simulink model "vehicle_suspension_model"  (R2015b)
settings: Solver=ode45  SolverMode=SingleTasking  StartTime=0.0  StopTime=10  MaxStep=0.01  RelTol=1e-3  AbsTol=1e-6
StopFcn:
  | if exist('sldemo_suspn_output')
  | sldemo_suspgraph
  | end
model workspace (MATLAB code in the model file):
  | sldemo_suspdat; %load data from file
undefined symbols (not defined in the file or in its folder): Iyy, Mb
undefined symbols (not defined in the file): cf, cr, kf, kr, Lf, Lr
CloseFcn:
  | if exist('suspnFigH')
  |   if ishghandle(suspnFigH,'figure')
  |     close(suspnFigH)
  |   end
  |   clear suspnFigH
  | end
  | if exist('suspnAxH'), clear suspnAxH; end
Description:
  | Automotive Suspension
  | 
  | This example shows how to model a simplified half-car model that includes an independent
  | front and rear vertical suspension. The model also includes body pitch and
  | bounce degrees of freedom. The example provides a description of the model to
  | show how simulation can be used for investigating ride characteristics.
  | In conjunction with a powertrain simulation, the model could
  | investigate longitudinal shuffle resulting from changes in throttle setting.
settings Model: ExtModeTrigMode=oneshot  ExtModeArmWhenConnect=off  ExtModeAutoUpdateStatusClock=off  Creator=The MathWorks, Inc.  LastModifiedBy=Samuel
settings DataIOCC: InitialState=x0  LimitDataPoints=off  SaveFormat=StructureWithTime  SaveOutput=off  SaveTime=off  StateSaveName=x  TimeSaveName=t  SignalLoggingName=sldemo_suspn_output
settings OptimizationCC: ExpressionDepthLimit=2147483647  InitFltsAndDblsToZero=on  BufferReusableBoundary=off
settings DebuggingCC: SaveWithParameterizedLinksMsg=none  UnderspecifiedInitializationDetection=Classic  MergeDetectMultiDrivingBlocksExec=none  SignalResolutionControl=TryResolveAllWithWarning  MultiTaskDSMMsg=warning  SigSpecEnsureSampleTimeMsg=none  IntegerOverflowMsg=none  FcnCallInpInsideContextMsg=UseLocalSettings  BusObjectLabelMismatch=none  StateNameClashWarn=warning  IntegerSaturationMsg=none
settings HardwareCC: ProdBitPerPointer=32  ProdLargestAtomicFloat=None  ProdIntDivRoundTo=Undefined  ProdEndianess=Unspecified  ProdWordSize=32  ProdHWDeviceType=32-bit Generic
settings GRTTargetCC: TargetFcnLib=ansi_tfl_tmw.mat  GeneratePreprocessorConditionals=Disable all  CombineOutputUpdateFcns=off  GRTInterface=on
settings ConfigComp: CovModelRefEnable=Off  CovSFcnEnable=off

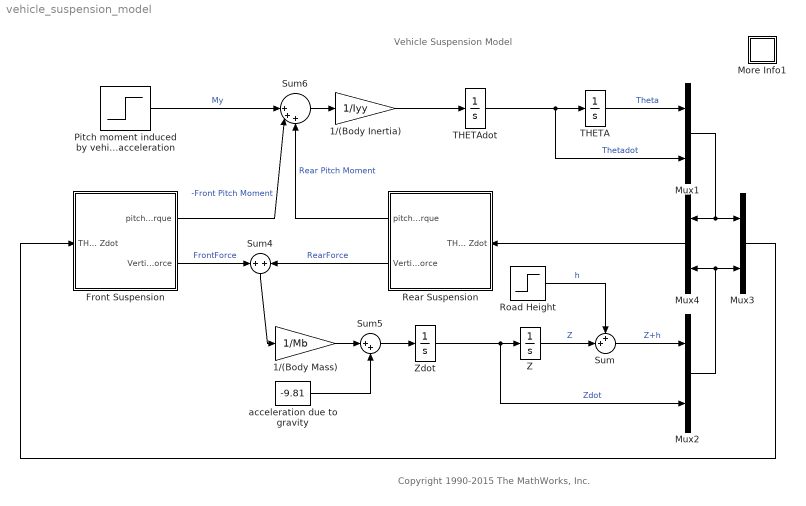
== system vehicle_suspension_model ==
  note: Vehicle Suspension Model
  note: Copyright 1990-2015 The MathWorks, Inc.
  1/(Body Inertia) : Gain  Gain=1/Iyy  SaturateOnIntegerOverflow=on  OutDataTypeStr=Inherit: Same as input  ParamDataTypeStr=Inherit: Same as input
  1/(Body Mass) : Gain  Gain=1/Mb  SaturateOnIntegerOverflow=on  OutDataTypeStr=Inherit: Same as input  ParamDataTypeStr=Inherit: Same as input
  Front Suspension : Subsystem  mask(half-car suspension){K=kf, C=cf, L=-Lf}
      mask prompts: K "Stiffness = spring rate:"; C "Damping rate:"; L "Moment arm:"
      mask help:
      | Half-Car Suspension
      | The spring and damping rates for an individual wheel are entered below.  Their combined effect as applied to two wheels at the specified distance from the center of mass is computed.  The distance should be specified as positive if the subsystem is oriented such that increasing z corresponds to increasing theta, negative otherwise.
      mask Help: See "Using Simulink and Stateflow in Automotive Applications" for a mathematical derivation of the subsystem operation.  Contact your MathWorks distributor to obtain a copy.
      mask Display: plot(-1, 0, 13, 12, [1 12], [11 11], [1 5], [2 2], [1 2], [4.5 5], [2 0], [5 6], [0 2], [6 7], [2 0], [7 8], [0 1], [8 8.5], [1 1], [8.5 11], [1 1], [2 4.5], [5 5], [2 5], [4 6], [5 5], [4 4], [5 8], [6 6], [5 8], [4 6], [6.5 6.5], [5 5], [6.5 11], [0 1], [1 2], [2 3], [1 2], [4 5], [1 2])
  More Info1 : Subsystem
      settings: OpenFcn=showdemo(bdroot(gcb))
      mask Display: disp('?')
  Mux{1..4} (4 alike) : Mux  Inputs=2
      settings: DisplayOption=signals
  Pitch moment induced by vehicle acceleration : Step  Time=3  After=100  SampleTime=0
  Rear Suspension : Subsystem  mask(half-car suspension){K=kr, C=cr, L=Lr}
      mask prompts: K "Stiffness = spring rate:"; C "Damping rate:"; L "Moment arm:"
      mask help:
      | Half-Car Suspension
      | The spring and damping rates for an individual wheel are entered below.  Their combined effect as applied to two wheels at the specified distance from the center of mass is computed.  The distance should be specified as positive if the subsystem is oriented such that increasing z corresponds to increasing theta, negative otherwise.
      mask Help: See "Using Simulink and Stateflow in Automotive Applications" for a mathematical derivation of the subsystem operation.  Contact your MathWorks distributor to obtain a copy.
      mask Display: plot(-1, 0, 13, 12, [1 12], [11 11], [1 5], [2 2], [1 2], [4.5 5], [2 0], [5 6], [0 2], [6 7], [2 0], [7 8], [0 1], [8 8.5], [1 1], [8.5 11], [1 1], [2 4.5], [5 5], [2 5], [4 6], [5 5], [4 4], [5 8], [6 6], [5 8], [4 6], [6.5 6.5], [5 5], [6.5 11], [0 1], [1 2], [2 3], [1 2], [4 5], [1 2])
  Road Height : Step  Time=7  After=0.01  SampleTime=0
  Sum : Sum  Inputs=++|
  Sum4 : Sum  SaturateOnIntegerOverflow=on  InputSameDT=on  OutDataTypeStr=Inherit: Same as first input
  Sum5 : Sum  Inputs=|++  SaturateOnIntegerOverflow=on  InputSameDT=on  OutDataTypeStr=Inherit: Same as first input
  Sum6 : Sum  Inputs=||+++  SaturateOnIntegerOverflow=on  InputSameDT=on  OutDataTypeStr=Inherit: Same as first input
  THETA : Integrator  InitialCondition=-8.7e-20
  THETAdot : Integrator  InitialCondition=8.04e-28
  Z : Integrator  InitialCondition=-0.12
  Zdot : Integrator
  acceleration due to gravity : Constant  Value=-9.81
  wires:
  Front Suspension/2(Vertical Force) -> Sum4/1  "FrontForce"
  Rear Suspension/2(Vertical Force) -> Sum4/2  "RearForce"
  Sum4/1 -> 1/(Body Mass)/1
  Mux1/1 -> Mux3/1, Mux4/1
  Mux3/1 -> Front Suspension/1(THETA THETAdot Z Zdot)
  Mux4/1 -> Rear Suspension/1(THETA THETAdot Z Zdot)
  Sum5/1 -> Zdot/1
  acceleration due to gravity/1 -> Sum5/2
  1/(Body Mass)/1 -> Sum5/1
  Zdot/1 -> Z/1, Mux2/2  "Zdot"
  Pitch moment induced by vehicle acceleration/1 -> Sum6/1  "My"
  Sum6/1 -> 1/(Body Inertia)/1
  Rear Suspension/1(pitch Torque) -> Sum6/3  "Rear Pitch Moment"
  Front Suspension/1(pitch Torque) -> Sum6/2  "-Front Pitch Moment"
  1/(Body Inertia)/1 -> THETAdot/1
  THETA/1 -> Mux1/1  "Theta"
  THETAdot/1 -> THETA/1, Mux1/2  "Thetadot"
  Mux2/1 -> Mux4/2, Mux3/2
  Road Height/1 -> Sum/1  "h"
  Z/1 -> Sum/2  "Z"
  Sum/1 -> Mux2/1  "Z+h"

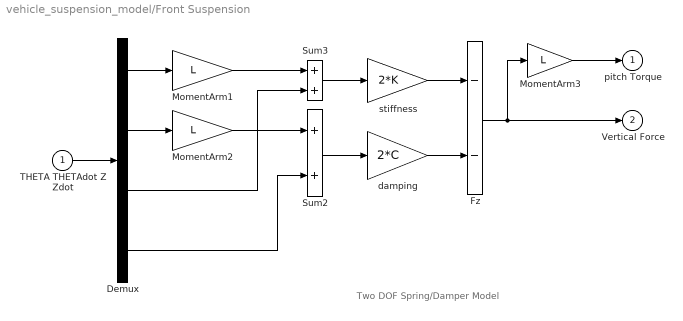
== system vehicle_suspension_model/Front Suspension ==
  note: Two DOF Spring/Damper Model
  THETA THETAdot Z Zdot : Inport
  Demux : Demux
  Fz : Sum  Inputs=--  SaturateOnIntegerOverflow=on  InputSameDT=on  OutDataTypeStr=Inherit: Same as first input
  MomentArm1 : Gain  Gain=L  SaturateOnIntegerOverflow=on  OutDataTypeStr=Inherit: Same as input  ParamDataTypeStr=Inherit: Same as input
  MomentArm2 : Gain  Gain=L  SaturateOnIntegerOverflow=on  OutDataTypeStr=Inherit: Same as input  ParamDataTypeStr=Inherit: Same as input
  MomentArm3 : Gain  Gain=L  SaturateOnIntegerOverflow=on  OutDataTypeStr=Inherit: Same as input  ParamDataTypeStr=Inherit: Same as input
  Sum2 : Sum  SaturateOnIntegerOverflow=on  InputSameDT=on  OutDataTypeStr=Inherit: Same as first input
  Sum3 : Sum  SaturateOnIntegerOverflow=on  InputSameDT=on  OutDataTypeStr=Inherit: Same as first input
  damping : Gain  Gain=2*C  SaturateOnIntegerOverflow=on  OutDataTypeStr=Inherit: Same as input  ParamDataTypeStr=Inherit: Same as input
  stiffness : Gain  Gain=2*K  SaturateOnIntegerOverflow=on  OutDataTypeStr=Inherit: Same as input  ParamDataTypeStr=Inherit: Same as input
  pitch Torque : Outport
  Vertical Force : Outport  Port=2
  wires:
  Sum2/1 -> damping/1
  Sum3/1 -> stiffness/1
  THETA THETAdot Z Zdot/1 -> Demux/1
  damping/1 -> Fz/2
  stiffness/1 -> Fz/1
  Fz/1 -> Vertical Force/1, MomentArm3/1
  MomentArm3/1 -> pitch Torque/1
  Demux/1 -> MomentArm1/1
  Demux/2 -> MomentArm2/1
  Demux/3 -> Sum3/2
  MomentArm1/1 -> Sum3/1
  MomentArm2/1 -> Sum2/1
  Demux/4 -> Sum2/2

== system vehicle_suspension_model/More Info1 ==

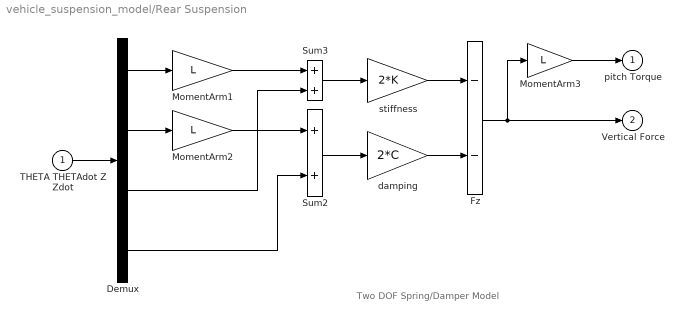
== system vehicle_suspension_model/Rear Suspension ==
  note: Two DOF Spring/Damper Model
  THETA THETAdot Z Zdot : Inport
  Demux : Demux
  Fz : Sum  Inputs=--  SaturateOnIntegerOverflow=on  InputSameDT=on  OutDataTypeStr=Inherit: Same as first input
  MomentArm1 : Gain  Gain=L  SaturateOnIntegerOverflow=on  OutDataTypeStr=Inherit: Same as input  ParamDataTypeStr=Inherit: Same as input
  MomentArm2 : Gain  Gain=L  SaturateOnIntegerOverflow=on  OutDataTypeStr=Inherit: Same as input  ParamDataTypeStr=Inherit: Same as input
  MomentArm3 : Gain  Gain=L  SaturateOnIntegerOverflow=on  OutDataTypeStr=Inherit: Same as input  ParamDataTypeStr=Inherit: Same as input
  Sum2 : Sum  SaturateOnIntegerOverflow=on  InputSameDT=on  OutDataTypeStr=Inherit: Same as first input
  Sum3 : Sum  SaturateOnIntegerOverflow=on  InputSameDT=on  OutDataTypeStr=Inherit: Same as first input
  damping : Gain  Gain=2*C  SaturateOnIntegerOverflow=on  OutDataTypeStr=Inherit: Same as input  ParamDataTypeStr=Inherit: Same as input
  stiffness : Gain  Gain=2*K  SaturateOnIntegerOverflow=on  OutDataTypeStr=Inherit: Same as input  ParamDataTypeStr=Inherit: Same as input
  pitch Torque : Outport
  Vertical Force : Outport  Port=2
  wires:
  Demux/4 -> Sum2/2
  MomentArm2/1 -> Sum2/1
  MomentArm1/1 -> Sum3/1
  Demux/3 -> Sum3/2
  Demux/2 -> MomentArm2/1
  Demux/1 -> MomentArm1/1
  MomentArm3/1 -> pitch Torque/1
  Fz/1 -> MomentArm3/1, Vertical Force/1
  stiffness/1 -> Fz/1
  damping/1 -> Fz/2
  THETA THETAdot Z Zdot/1 -> Demux/1
  Sum3/1 -> stiffness/1
  Sum2/1 -> damping/1
